simulink model "controller_estimator_minimal"  (R2016b)
settings: Solver=VariableStepAuto  StartTime=0.0  StopTime=100  RelTol=1e-3
undefined symbols (not defined in the file or in its folder): quat_init, sim_params
libraries: dynamics_lib x2, pd_control_lib x1, RW_assembly_simple_lib x1, extended_kalman_filter_lib x1
settings Model: Creator=sexymathemagician  LastModifiedBy=sexymathemagician

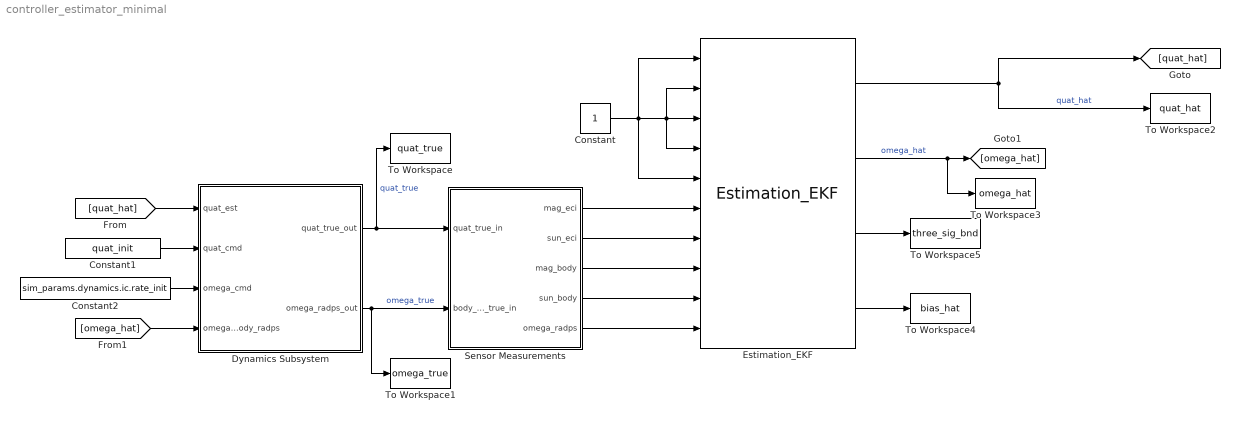
== system controller_estimator_minimal ==
  Constant : Constant
  Constant1 : Constant  Value=quat_init
  Constant2 : Constant  Value=sim_params.dynamics.ic.rate_init
  Dynamics Subsystem : Subsystem
  "Estimation_EKF " : extended_kalman_filter_lib/Estimation_EKF 
  "Sensor Measurements " : Subsystem
  To Workspace : ToWorkspace  VariableName=quat_true  SaveFormat=Timeseries  SampleTime=-1
  To Workspace1 : ToWorkspace  VariableName=omega_true  SaveFormat=Timeseries  SampleTime=-1
  To Workspace2 : ToWorkspace  VariableName=quat_hat  SaveFormat=Timeseries  SampleTime=-1
  To Workspace3 : ToWorkspace  VariableName=omega_hat  SaveFormat=Timeseries  SampleTime=-1
  To Workspace4 : ToWorkspace  VariableName=bias_hat  SaveFormat=Timeseries  SampleTime=-1
  To Workspace5 : ToWorkspace  VariableName=three_sig_bnd  SaveFormat=Timeseries  SampleTime=-1
  wires:
  "Sensor Measurements "/1(mag_eci) -> "Estimation_EKF "/6
  "Sensor Measurements "/2(sun_eci) -> "Estimation_EKF "/7
  "Sensor Measurements "/3(mag_body) -> "Estimation_EKF "/8
  "Sensor Measurements "/4(sun_body) -> "Estimation_EKF "/9
  Constant/1 -> "Estimation_EKF "/5, "Estimation_EKF "/1, "Estimation_EKF "/4, "Estimation_EKF "/2, "Estimation_EKF "/3
  "Estimation_EKF "/3 -> To Workspace5/1
  "Estimation_EKF "/4 -> To Workspace4/1
  Dynamics Subsystem/1(quat_true_out) -> To Workspace/1, "Sensor Measurements "/1(quat_true_in)  "quat_true"
  Dynamics Subsystem/2(omega_radps_out) -> To Workspace1/1, "Sensor Measurements "/2(body_rates_true_in)  "omega_true"
  "Sensor Measurements "/5(omega_radps) -> "Estimation_EKF "/10
  [quat_hat] -> Dynamics Subsystem/1(quat_est)
  "Estimation_EKF "/2 -> To Workspace3/1, [omega_hat]  "omega_hat"
  [omega_hat] -> Dynamics Subsystem/4(omega_body_radps)
  Constant1/1 -> Dynamics Subsystem/2(quat_cmd)
  Constant2/1 -> Dynamics Subsystem/3("omega_cmd ")
  "Estimation_EKF "/1 -> To Workspace2/1, [quat_hat]  "quat_hat"

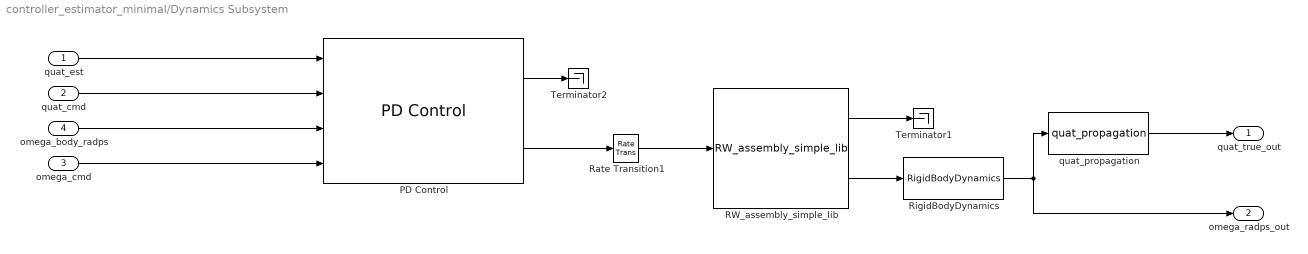
== system controller_estimator_minimal/Dynamics Subsystem ==
  quat_est : Inport
  quat_cmd : Inport  Port=2
  "omega_cmd " : Inport  Port=3
  omega_body_radps : Inport  Port=4
  PD Control : pd_control_lib/PD Control
  RW_assembly_simple_lib : RW_assembly_simple_lib/RW_assembly_simple_lib  natural_frequency=sim_params.actuators.reaction_wheel.natural_freq  damping_ratio=sim_params.actuators.reaction_wheel.damping  max_rate=sim_params.actuators.reaction_wheel.rate_limit
  Rate Transition1 : RateTransition  OutPortSampleTime=1/20
  RigidBodyDynamics : dynamics_lib/Dynamics/RigidBodyDynamics
  Terminator1 : Terminator
  Terminator2 : Terminator
  quat_propagation : dynamics_lib/Dynamics/quat_propagation
  quat_true_out : Outport
  omega_radps_out : Outport  Port=2
  wires:
  "omega_cmd "/1 -> PD Control/4
  quat_est/1 -> PD Control/1
  quat_cmd/1 -> PD Control/2
  omega_body_radps/1 -> PD Control/3
  PD Control/2 -> Rate Transition1/1
  Rate Transition1/1 -> RW_assembly_simple_lib/1
  RW_assembly_simple_lib/1 -> Terminator1/1
  RigidBodyDynamics/1 -> omega_radps_out/1, quat_propagation/1
  RW_assembly_simple_lib/2 -> RigidBodyDynamics/1
  quat_propagation/1 -> quat_true_out/1
  PD Control/1 -> Terminator2/1

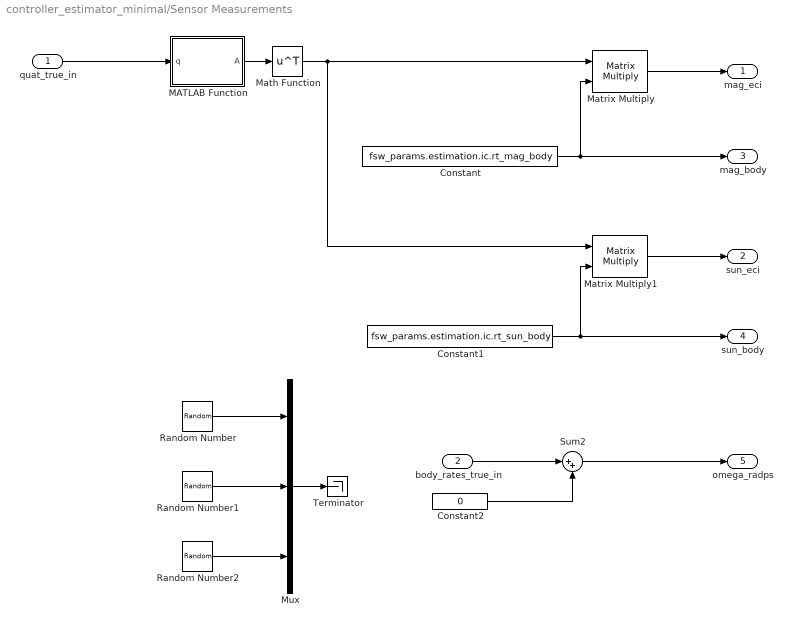
== system controller_estimator_minimal/Sensor Measurements  ==
  quat_true_in : Inport
  body_rates_true_in : Inport  Port=2
  Constant : Constant  Value=fsw_params.estimation.ic.rt_mag_body
  Constant1 : Constant  Value=fsw_params.estimation.ic.rt_sun_body
  Constant2 : Constant  Value=0
  MATLAB Function : MATLAB Function  TreatAsAtomicUnit=on
  Math Function : Math  Operator=transpose  SaturateOnIntegerOverflow=on
  Matrix Multiply : Product  Multiplication=Matrix(*)
  Matrix Multiply1 : Product  Multiplication=Matrix(*)
  Mux : Mux  Inputs=3
  Random Number : RandomNumber  Variance=(sim_params.sensors.gyro.arw)^2/(60*60)  SampleTime=0.1
  Random Number1 : RandomNumber  Variance=(sim_params.sensors.gyro.arw)^2/(60*60)  SampleTime=0.1
  Random Number2 : RandomNumber  Variance=(sim_params.sensors.gyro.arw)^2/(60*60)  SampleTime=0.1
  Sum2 : Sum  Inputs=|++
  Terminator : Terminator
  mag_eci : Outport
  sun_eci : Outport  Port=2
  mag_body : Outport  Port=3
  sun_body : Outport  Port=4
  omega_radps : Outport  Port=5
  wires:
  quat_true_in/1 -> MATLAB Function/1(q)
  Constant/1 -> Matrix Multiply/2, mag_body/1
  Matrix Multiply/1 -> mag_eci/1
  Constant1/1 -> Matrix Multiply1/2, sun_body/1
  Matrix Multiply1/1 -> sun_eci/1
  Random Number/1 -> Mux/1
  Random Number1/1 -> Mux/2
  Random Number2/1 -> Mux/3
  body_rates_true_in/1 -> Sum2/1
  Sum2/1 -> omega_radps/1
  Mux/1 -> Terminator/1
  Constant2/1 -> Sum2/2
  MATLAB Function/1(A) -> Math Function/1
  Math Function/1 -> Matrix Multiply1/1, Matrix Multiply/1

== matlab function controller_estimator_minimal/Sensor Measurements /MATLAB Function ==
  data: q input; A output
function A = quatToMatrix(q)
%#codegen

eta = q(1);
eps = q(2:4);

A = (2*eta^2 -1)*eye(3) + 2*(eps*eps') - 2*eta*skew(eps);


end

function cross = skew(a)
%#codegen

cross = [0 -a(3) a(2);
         a(3) 0 -a(1);
        -a(2) a(1) 0];

end
